simulink model "EPD629_WilliamsJ_AS12"  (R2021b)
settings: Solver=VariableStepAuto  StartTime=0.0  StopTime=45  MaxStep=0.0005  RelTol=1e-3
values from neighbouring files (symbols this model uses):
  AirMassFracO2 = 0.233    [EPD629_HW12_init.m]
  BPVAreaBreakpoints_pct = BPVAreaData_pct    [EPD629_HW12_init.m]
  BPVAreaData_pct = EGRValveAreaData_pct    [EPD629_HW12_init.m]
  BPVPositionBreakpoints_pct = EGRValvePositionBreakpoints_pct    [EPD629_HW12_init.m]
  BPVPositionData_pct = BPVPositionBreakpoints_pct    [EPD629_HW12_init.m]
  BPVWideOpenArea_mm2 = pi * BPVDiameter_mm^2 / 4    (= 7853.98163397)    [EPD629_HW12_init.m]
  CACDischargeCoefficient_frac = 0.7    [EPD629_HW12_init.m]
  CACEffectivenessData_frac = [1 0.95 0.92 0.885 0.87 0.85]    [EPD629_HW12_init.m]
  CACEffectivenessMassFlowBP_gps = [0 50 100 200 300 500]    [EPD629_HW12_init.m]
  CACFlowRestrictionArea_mm2 = 2000    [EPD629_HW12_init.m]
  CACVolume_L = 40    [EPD629_HW12_init.m]
  ClearanceVolumeTotal_L = 8/15    (= 0.533333333333)    [EPD629_HW12_init.m]
  Cp_cmp = 1.004    [EPD629_HW12_init.m]
  Cp_trb = 1.073    [EPD629_HW12_init.m]
  DesiredFuelBreakpoints_mg = 0:20:500    [EPD629_HW12_init.m]
  DischargeCoefficient_frac = 0.7    [EPD629_HW12_init.m]
  EGRCDischargeCoefficient_frac = 0.7    [EPD629_HW12_init.m]
  EGRCEffectivenessData_frac = [1 0.95 0.92 0.885 0.87 0.85]    [EPD629_HW12_init.m]
  EGRCEffectivenessMassFlowBP_gps = [0 50 100 200 300 500]    [EPD629_HW12_init.m]
  EGRCFlowRestrictionArea_mm2 = 500    [EPD629_HW12_init.m]
  EGRCoolerToValveVolume_L = 2    [EPD629_HW12_init.m]
  EGRValveAreaBreakpoints_pct = EGRValveAreaData_pct    [EPD629_HW12_init.m]
  EGRValveAreaData_pct = 100 * EGRValveArea_mm2 / EGRValveWideOpenArea_mm2    [EPD629_HW12_init.m]
  EGRValvePositionBreakpoints_pct = 0:100    [EPD629_HW12_init.m]
  EGRValvePositionData_pct = EGRValvePositionBreakpoints_pct    [EPD629_HW12_init.m]
  EGRValveWideOpenArea_mm2 = pi/4*50^2    (= 1963.49540849)    [EPD629_HW12_init.m]
  EngineDisplacement_L = 8    [EPD629_HW12_init.m]
  EngineSpeedBreakpoints_rpm = 600:200:3000    [EPD629_HW12_init.m]
  ExhaustManifoldGasConstant_kJpkgK = R_trb    (= 0.287)    [EPD629_HW12_init.m]
  ExhaustManifoldVolume_L = 8    [EPD629_HW12_init.m]
  FlowFunctionData_frac = PR.^(1/k_trb) .*      sqrt( 2 * k_trb / (k_trb - 1) .*      (1 - PR.^((k_trb - 1) / k_trb)) )    [EPD629_HW12_init.m]
  IntakeManifoldGasConstant_kJpkgK = Cp_im - Cv_im    (= 0.288)    [EPD629_HW12_init.m]
  IntakeManifoldVolume_L = 8    [EPD629_HW12_init.m]
  k_cmp = Cp_cmp/Cv_cmp    (= 1.40027894003)    [EPD629_HW12_init.m]
  k_trb = Cp_trb/Cv_trb    (= 1.36513994911)    [EPD629_HW12_init.m]
  ManifoldPressureBreakpoints_kPa = 80:20:500    [EPD629_HW12_init.m]
  NumberOfCylinders = 6    [EPD629_HW12_init.m]
  PressureRatioBreakpoints_frac = 0:0.01:1    [EPD629_HW12_init.m]
  R_cmp = Cp_cmp - Cv_cmp    (= 0.287)    [EPD629_HW12_init.m]
  R_trb = Cp_trb - Cv_trb    (= 0.287)    [EPD629_HW12_init.m]
  StoichiometricAFR_frac = 14.7    [EPD629_HW12_init.m]
  TurbineToBPVVolume_L = 10    [EPD629_HW12_init.m]
  TurbochargerInertia_kgm2 = 1e-4    (= 0.0001)    [EPD629_HW12_init.m]
  WastegateAreaData_pct = [0 100]    [EPD629_HW12_init.m]
  WastegateAreaGagePressBreakpoints_kPa = [250 300]    [EPD629_HW12_init.m]
  WastegateWideOpenArea_mm2 = pi/4*20^2    (= 314.159265359)    [EPD629_HW12_init.m]
undefined symbols (not defined in the file or in its folder): APPR_cmp, APPR_trb, ARPM_cmp, ARPM_trb, EFFI_cmp, EFFI_trb, ExhaustTemperatureData_degC, MASS_cmp, MASS_trb, MXRSP_cmp, MXRSP_trb, MXRVOL_cmp, MXRVOL_trb, PMAX_cmp, PMAX_trb, PMIN_cmp, PMIN_trb, ResidualCorrectionFactorData, VolumetricEfficiencyData_frac
libraries: simulink x2
(part 2 of 3)

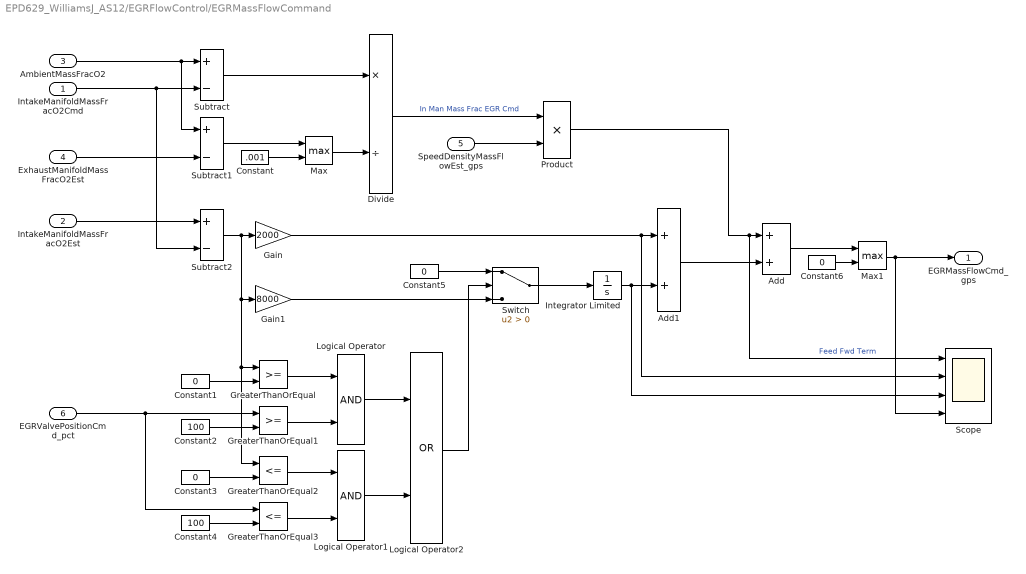
== system EPD629_WilliamsJ_AS12/EGRFlowControl/EGRMassFlowCommand ==
  IntakeManifoldMassFracO2Cmd : Inport
  IntakeManifoldMassFracO2Est : Inport  Port=2
  AmbientMassFracO2 : Inport  Port=3
  ExhaustManifoldMassFracO2Est : Inport  Port=4
  SpeedDensityMassFlowEst_gps : Inport  Port=5
  EGRValvePositionCmd_pct : Inport  Port=6
  Add : Sum
  Add1 : Sum
  Constant : Constant  Value=.001
  Constant{1,3,5..6} (4 alike) : Constant  Value=0
  Constant2 : Constant  Value=100
  Constant4 : Constant  Value=100
  Divide : Product  Inputs=*/
  Gain : Gain  Gain=2000
  Gain1 : Gain  Gain=8000
  GreaterThanOrEqual : RelationalOperator  OutDataTypeStr=boolean  RndMeth=Simplest
  GreaterThanOrEqual1 : RelationalOperator  OutDataTypeStr=boolean  RndMeth=Simplest
  GreaterThanOrEqual2 : RelationalOperator  Operator=<=  OutDataTypeStr=boolean  RndMeth=Simplest
  GreaterThanOrEqual3 : RelationalOperator  Operator=<=  OutDataTypeStr=boolean  RndMeth=Simplest
  Integrator Limited : Integrator  LimitOutput=on  UpperSaturationLimit=20  LowerSaturationLimit=-20
  Logical Operator : Logic  AllPortsSameDT=off  OutDataTypeStr=boolean
  Logical Operator1 : Logic  AllPortsSameDT=off  OutDataTypeStr=boolean
  Logical Operator2 : Logic  Operator=OR  AllPortsSameDT=off  OutDataTypeStr=boolean
  Max : MinMax  Function=max  Inputs=2
  Max1 : MinMax  Function=max  Inputs=2
  Product : Product
  Scope : Scope  NumInputPorts=4
  Subtract : Sum  Inputs=+-
  Subtract1 : Sum  Inputs=+-
  Subtract2 : Sum  Inputs=+-
  Switch : Switch  Criteria=u2 > Threshold
  EGRMassFlowCmd_gps : Outport
  wires:
  AmbientMassFracO2/1 -> Subtract/1, Subtract1/1
  IntakeManifoldMassFracO2Cmd/1 -> Subtract2/2, Subtract/2
  ExhaustManifoldMassFracO2Est/1 -> Subtract1/2
  IntakeManifoldMassFracO2Est/1 -> Subtract2/1
  Constant/1 -> Max/2
  Subtract1/1 -> Max/1
  Subtract/1 -> Divide/1
  Max/1 -> Divide/2
  Divide/1 -> Product/1  "In Man Mass Frac EGR Cmd"
  SpeedDensityMassFlowEst_gps/1 -> Product/2
  Product/1 -> Scope/1, Add/1  "Feed Fwd Term"
  Subtract2/1 -> GreaterThanOrEqual2/1, GreaterThanOrEqual/1, Gain1/1, Gain/1
  Gain/1 -> Scope/2, Add1/1
  Gain1/1 -> Switch/3
  Constant1/1 -> GreaterThanOrEqual/2
  EGRValvePositionCmd_pct/1 -> GreaterThanOrEqual3/1, GreaterThanOrEqual1/1
  Constant2/1 -> GreaterThanOrEqual1/2
  Constant3/1 -> GreaterThanOrEqual2/2
  Constant4/1 -> GreaterThanOrEqual3/2
  GreaterThanOrEqual1/1 -> Logical Operator/2
  GreaterThanOrEqual/1 -> Logical Operator/1
  GreaterThanOrEqual2/1 -> Logical Operator1/1
  GreaterThanOrEqual3/1 -> Logical Operator1/2
  Logical Operator/1 -> Logical Operator2/1
  Logical Operator1/1 -> Logical Operator2/2
  Constant5/1 -> Switch/1
  Logical Operator2/1 -> Switch/2
  Switch/1 -> Integrator Limited/1
  Integrator Limited/1 -> Scope/3, Add1/2
  Add1/1 -> Add/2
  Constant6/1 -> Max1/2
  Add/1 -> Max1/1
  Max1/1 -> Scope/4, EGRMassFlowCmd_gps/1

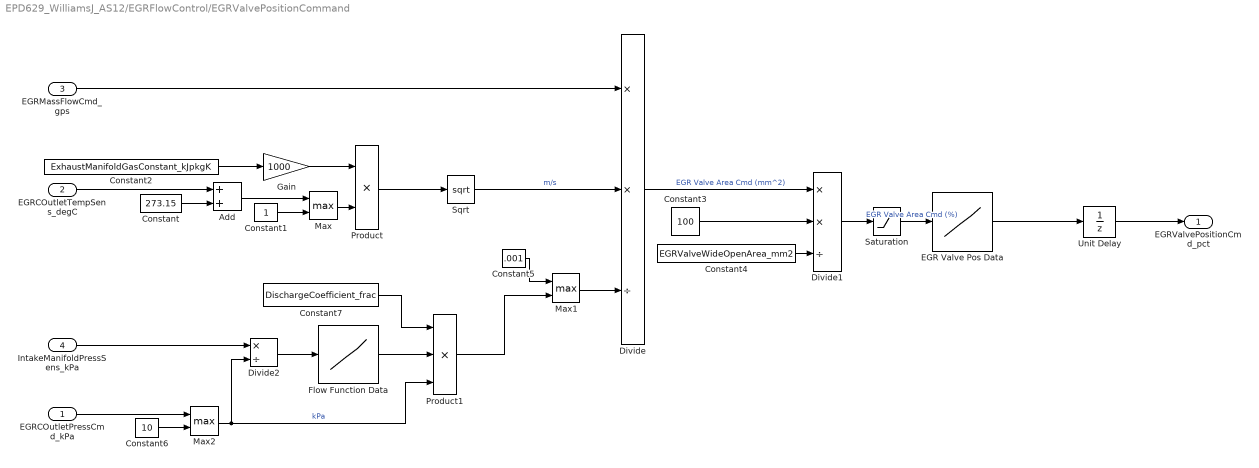
== system EPD629_WilliamsJ_AS12/EGRFlowControl/EGRValvePositionCommand ==
  EGRCOutletPressCmd_kPa : Inport
  EGRCOutletTempSens_degC : Inport  Port=2
  EGRMassFlowCmd_gps : Inport  Port=3
  IntakeManifoldPressSens_kPa : Inport  Port=4
  Add : Sum
  Constant : Constant  Value=273.15
  Constant1 : Constant
  Constant2 : Constant  Value=ExhaustManifoldGasConstant_kJpkgK
  Constant3 : Constant  Value=100
  Constant4 : Constant  Value=EGRValveWideOpenArea_mm2
  Constant5 : Constant  Value=.001
  Constant6 : Constant  Value=10
  Constant7 : Constant  Value=DischargeCoefficient_frac
  Divide : Product  Inputs=**/
  Divide1 : Product  Inputs=**/
  Divide2 : Product  Inputs=*/
  EGR Valve Pos Data : Lookup_n-D  NumberOfTableDimensions=1  BreakpointsForDimension1=EGRValveAreaBreakpoints_pct  Table=EGRValvePositionData_pct  ExtrapMethod=Clip  UseLastTableValue=on  InternalRulePriority=Speed  RndMeth=Simplest  InputSameDT=on
  Flow Function Data : Lookup_n-D  NumberOfTableDimensions=1  BreakpointsForDimension1=PressureRatioBreakpoints_frac  Table=FlowFunctionData_frac  ExtrapMethod=Clip  UseLastTableValue=on  InternalRulePriority=Speed  RndMeth=Simplest  InputSameDT=on
  Gain : Gain  Gain=1000
  Max : MinMax  Function=max  Inputs=2
  Max1 : MinMax  Function=max  Inputs=2
  Max2 : MinMax  Function=max  Inputs=2
  Product : Product
  Product1 : Product  Inputs=3
  Saturation : Saturate  UpperLimit=100  LowerLimit=0
  Sqrt : Sqrt  SaturateOnIntegerOverflow=on
  Unit Delay : UnitDelay  SampleTime=-1  HasFrameUpgradeWarning=on
      settings: AttributesFormatString=IC: %<InitialCondition>
  EGRValvePositionCmd_pct : Outport
  wires:
  Unit Delay/1 -> EGRValvePositionCmd_pct/1
  Constant/1 -> Add/2
  EGRCOutletTempSens_degC/1 -> Add/1
  Add/1 -> Max/1
  Constant1/1 -> Max/2
  Max/1 -> Product/2
  Gain/1 -> Product/1
  Constant2/1 -> Gain/1
  EGRMassFlowCmd_gps/1 -> Divide/1
  Product/1 -> Sqrt/1
  Sqrt/1 -> Divide/2  "m/s"
  Divide/1 -> Divide1/1  "EGR Valve Area Cmd (mm^2)"
  Constant3/1 -> Divide1/2
  Constant4/1 -> Divide1/3
  Divide1/1 -> Saturation/1
  Saturation/1 -> EGR Valve Pos Data/1  "EGR Valve Area Cmd (%)"
  EGR Valve Pos Data/1 -> Unit Delay/1
  Constant5/1 -> Max1/1
  Max1/1 -> Divide/3
  IntakeManifoldPressSens_kPa/1 -> Divide2/1
  Constant6/1 -> Max2/2
  EGRCOutletPressCmd_kPa/1 -> Max2/1
  Max2/1 -> Divide2/2, Product1/3  "kPa"
  Divide2/1 -> Flow Function Data/1
  Flow Function Data/1 -> Product1/2
  Constant7/1 -> Product1/1
  Product1/1 -> Max1/2

== system EPD629_WilliamsJ_AS12/EGRFlowControl/IntakeManifoldMassFractionO2Command ==
  CylinderInMassEst_mg : Inport
  CylinderIVCMassEst_mg : Inport  Port=2
  CylinderIVCMassFracO2Cmd : Inport  Port=3
  CylinderResidualMassO2Est_mg : Inport  Port=4
  Constant : Constant  Value=0
  Constant1 : Constant
  Divide : Product  Inputs=*/
  Max : MinMax  Function=max  Inputs=2
  Max1 : MinMax  Function=max  Inputs=2
  Product : Product
  Subtract : Sum  Inputs=+-
  IntakeManifoldMassFracO2Cmd : Outport
  wires:
  CylinderIVCMassFracO2Cmd/1 -> Product/1
  CylinderIVCMassEst_mg/1 -> Product/2
  Product/1 -> Subtract/1  "Cyl IVC Mass O2 Cmd (mg)"
  CylinderResidualMassO2Est_mg/1 -> Subtract/2
  Subtract/1 -> Max/2
  Constant/1 -> Max/1
  Max/1 -> Divide/1  "Cyl In Mass O2 Cmd (mg)"
  Constant1/1 -> Max1/2
  CylinderInMassEst_mg/1 -> Max1/1
  Max1/1 -> Divide/2
  Divide/1 -> IntakeManifoldMassFracO2Cmd/1

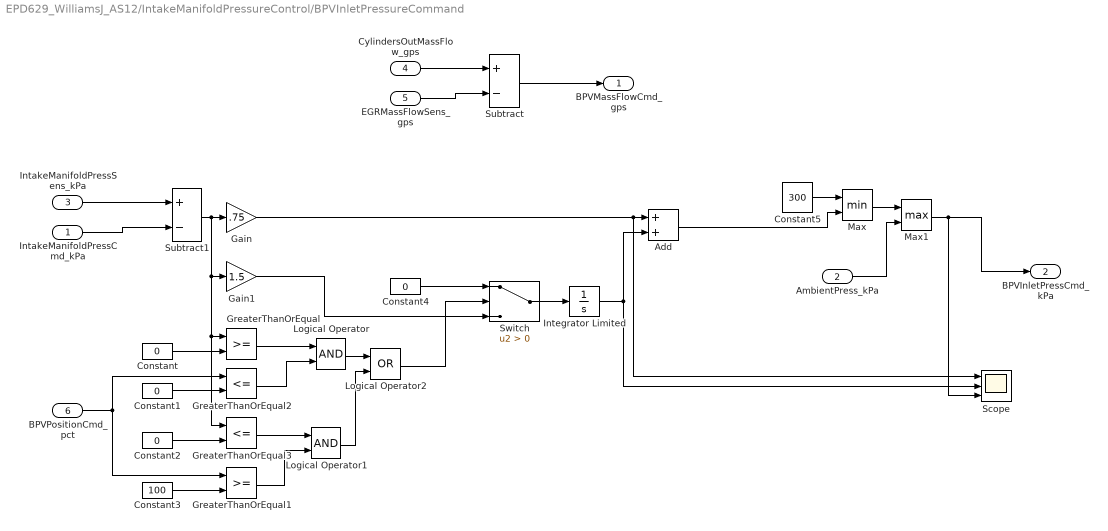
== system EPD629_WilliamsJ_AS12/IntakeManifoldPressureControl/BPVInletPressureCommand ==
  IntakeManifoldPressCmd_kPa : Inport
  AmbientPress_kPa : Inport  Port=2
  IntakeManifoldPressSens_kPa : Inport  Port=3
  CylindersOutMassFlow_gps : Inport  Port=4
  EGRMassFlowSens_gps : Inport  Port=5
  BPVPositionCmd_pct : Inport  Port=6
  Add : Sum
  Constant{,1..2,4} (4 alike) : Constant  Value=0
  Constant3 : Constant  Value=100
  Constant5 : Constant  Value=300
  Gain : Gain  Gain=.75
  Gain1 : Gain  Gain=1.5
  GreaterThanOrEqual : RelationalOperator  OutDataTypeStr=boolean  RndMeth=Simplest
  GreaterThanOrEqual1 : RelationalOperator  OutDataTypeStr=boolean  RndMeth=Simplest
  GreaterThanOrEqual2 : RelationalOperator  Operator=<=  OutDataTypeStr=boolean  RndMeth=Simplest
  GreaterThanOrEqual3 : RelationalOperator  Operator=<=  OutDataTypeStr=boolean  RndMeth=Simplest
  Integrator Limited : Integrator  InitialCondition=100  LimitOutput=on  UpperSaturationLimit=300  LowerSaturationLimit=100
  Logical Operator : Logic  AllPortsSameDT=off  OutDataTypeStr=boolean
  Logical Operator1 : Logic  AllPortsSameDT=off  OutDataTypeStr=boolean
  Logical Operator2 : Logic  Operator=OR  AllPortsSameDT=off  OutDataTypeStr=boolean
  Max : MinMax  Inputs=2
  Max1 : MinMax  Function=max  Inputs=2
  Scope : Scope  NumInputPorts=3
  Subtract : Sum  Inputs=+-
  Subtract1 : Sum  Inputs=+-
  Switch : Switch  Criteria=u2 > Threshold
  BPVMassFlowCmd_gps : Outport
  BPVInletPressCmd_kPa : Outport  Port=2
  wires:
  CylindersOutMassFlow_gps/1 -> Subtract/1
  EGRMassFlowSens_gps/1 -> Subtract/2
  Subtract/1 -> BPVMassFlowCmd_gps/1
  IntakeManifoldPressSens_kPa/1 -> Subtract1/1
  IntakeManifoldPressCmd_kPa/1 -> Subtract1/2
  Subtract1/1 -> GreaterThanOrEqual3/1, GreaterThanOrEqual/1, Gain1/1, Gain/1
  Gain/1 -> Scope/1, Add/1
  Constant/1 -> GreaterThanOrEqual/2
  Constant1/1 -> GreaterThanOrEqual2/2
  BPVPositionCmd_pct/1 -> GreaterThanOrEqual1/1, GreaterThanOrEqual2/1
  Constant2/1 -> GreaterThanOrEqual3/2
  Constant3/1 -> GreaterThanOrEqual1/2
  GreaterThanOrEqual/1 -> Logical Operator/1
  GreaterThanOrEqual2/1 -> Logical Operator/2
  GreaterThanOrEqual3/1 -> Logical Operator1/1
  GreaterThanOrEqual1/1 -> Logical Operator1/2
  Logical Operator/1 -> Logical Operator2/1
  Logical Operator1/1 -> Logical Operator2/2
  Constant4/1 -> Switch/1
  Logical Operator2/1 -> Switch/2
  Gain1/1 -> Switch/3
  Switch/1 -> Integrator Limited/1
  Integrator Limited/1 -> Add/2, Scope/2
  Constant5/1 -> Max/1
  Add/1 -> Max/2
  Max/1 -> Max1/1
  AmbientPress_kPa/1 -> Max1/2
  Max1/1 -> Scope/3, BPVInletPressCmd_kPa/1

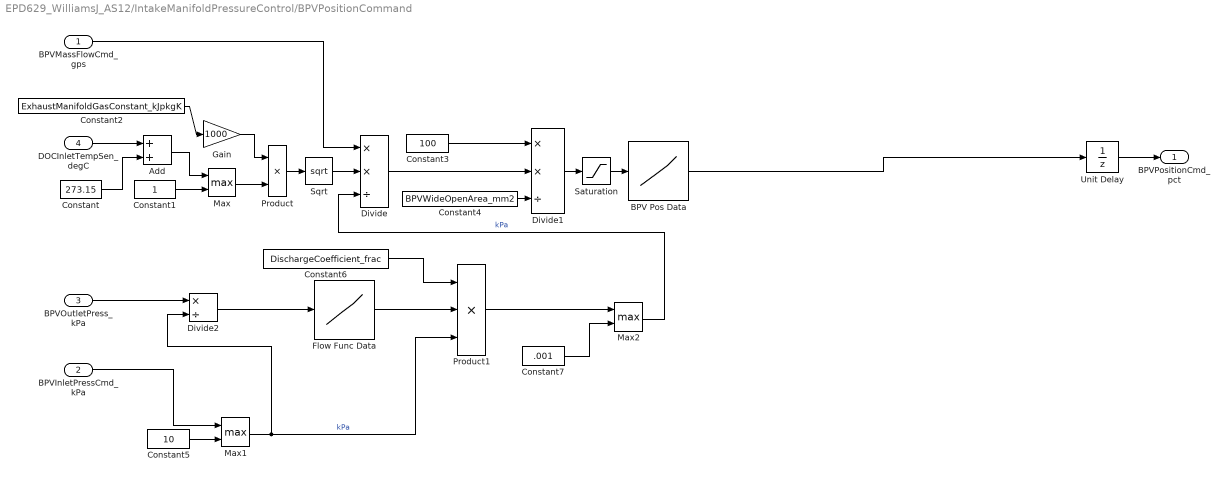
== system EPD629_WilliamsJ_AS12/IntakeManifoldPressureControl/BPVPositionCommand ==
  BPVMassFlowCmd_gps : Inport
  BPVInletPressCmd_kPa : Inport  Port=2
  BPVOutletPress_kPa : Inport  Port=3
  DOCInletTempSen_degC : Inport  Port=4
  Add : Sum
  BPV Pos Data : Lookup_n-D  NumberOfTableDimensions=1  BreakpointsForDimension1=BPVAreaBreakpoints_pct  Table=BPVPositionData_pct  ExtrapMethod=Clip  UseLastTableValue=on  InternalRulePriority=Speed  RndMeth=Simplest  InputSameDT=on
  Constant : Constant  Value=273.15
  Constant1 : Constant
  Constant2 : Constant  Value=ExhaustManifoldGasConstant_kJpkgK
  Constant3 : Constant  Value=100
  Constant4 : Constant  Value=BPVWideOpenArea_mm2
  Constant5 : Constant  Value=10
  Constant6 : Constant  Value=DischargeCoefficient_frac
  Constant7 : Constant  Value=.001
  Divide : Product  Inputs=**/
  Divide1 : Product  Inputs=**/
  Divide2 : Product  Inputs=*/
  Flow Func Data : Lookup_n-D  NumberOfTableDimensions=1  BreakpointsForDimension1=PressureRatioBreakpoints_frac  Table=FlowFunctionData_frac  ExtrapMethod=Clip  UseLastTableValue=on  InternalRulePriority=Speed  RndMeth=Simplest  InputSameDT=on
  Gain : Gain  Gain=1000
  Max : MinMax  Function=max  Inputs=2
  Max1 : MinMax  Function=max  Inputs=2
  Max2 : MinMax  Function=max  Inputs=2
  Product : Product
  Product1 : Product  Inputs=3
  Saturation : Saturate  UpperLimit=100  LowerLimit=0
  Sqrt : Sqrt  SaturateOnIntegerOverflow=on
  Unit Delay : UnitDelay  InitialCondition=100  SampleTime=-1  HasFrameUpgradeWarning=on
      settings: AttributesFormatString=IC: %<InitialCondition>
  BPVPositionCmd_pct : Outport
  wires:
  Unit Delay/1 -> BPVPositionCmd_pct/1
  DOCInletTempSen_degC/1 -> Add/1
  Constant/1 -> Add/2
  Constant1/1 -> Max/2
  Add/1 -> Max/1
  Max/1 -> Product/2
  Gain/1 -> Product/1
  Constant2/1 -> Gain/1
  Product/1 -> Sqrt/1
  Sqrt/1 -> Divide/2
  BPVMassFlowCmd_gps/1 -> Divide/1
  Divide/1 -> Divide1/2
  Constant3/1 -> Divide1/1
  Constant4/1 -> Divide1/3
  Divide1/1 -> Saturation/1
  Saturation/1 -> BPV Pos Data/1
  BPV Pos Data/1 -> Unit Delay/1
  Max1/1 -> Product1/3, Divide2/2  "kPa"
  Constant5/1 -> Max1/2
  BPVInletPressCmd_kPa/1 -> Max1/1
  BPVOutletPress_kPa/1 -> Divide2/1
  Divide2/1 -> Flow Func Data/1
  Flow Func Data/1 -> Product1/2
  Constant6/1 -> Product1/1
  Constant7/1 -> Max2/2
  Product1/1 -> Max2/1
  Max2/1 -> Divide/3  "kPa"

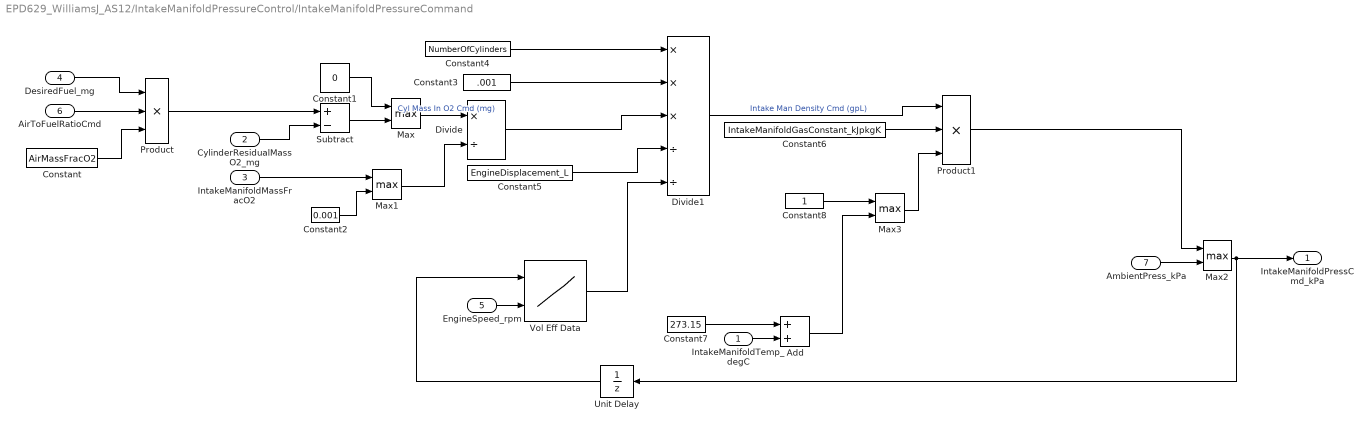
== system EPD629_WilliamsJ_AS12/IntakeManifoldPressureControl/IntakeManifoldPressureCommand ==
  IntakeManifoldTemp_degC : Inport
  CylinderResidualMassO2_mg : Inport  Port=2
  IntakeManifoldMassFracO2 : Inport  Port=3
  DesiredFuel_mg : Inport  Port=4
  EngineSpeed_rpm : Inport  Port=5
  AirToFuelRatioCmd : Inport  Port=6
  AmbientPress_kPa : Inport  Port=7
  Add : Sum
  Constant : Constant  Value=AirMassFracO2
  Constant1 : Constant  Value=0
  Constant2 : Constant  Value=0.001
  Constant3 : Constant  Value=.001
  Constant4 : Constant  Value=NumberOfCylinders
  Constant5 : Constant  Value=EngineDisplacement_L
  Constant6 : Constant  Value=IntakeManifoldGasConstant_kJpkgK
  Constant7 : Constant  Value=273.15
  Constant8 : Constant
  Divide : Product  Inputs=*/
  Divide1 : Product  Inputs=***//
  Max{,1..3} (4 alike) : MinMax  Function=max  Inputs=2
  Product : Product  Inputs=3
  Product1 : Product  Inputs=3
  Subtract : Sum  Inputs=+-
  Unit Delay : UnitDelay  InitialCondition=100  SampleTime=-1  HasFrameUpgradeWarning=on
  Vol Eff Data : Lookup_n-D  BreakpointsForDimension1=ManifoldPressureBreakpoints_kPa  BreakpointsForDimension2=EngineSpeedBreakpoints_rpm  Table=VolumetricEfficiencyData_frac  ExtrapMethod=Clip  UseLastTableValue=on  InternalRulePriority=Speed  RndMeth=Simplest  InputSameDT=on
      settings: InputPortMap=u0,u1
  IntakeManifoldPressCmd_kPa : Outport
  wires:
  DesiredFuel_mg/1 -> Product/1
  AirToFuelRatioCmd/1 -> Product/2
  Constant/1 -> Product/3
  Product/1 -> Subtract/1
  CylinderResidualMassO2_mg/1 -> Subtract/2
  Subtract/1 -> Max/2
  Constant1/1 -> Max/1
  Max/1 -> Divide/1  "Cyl Mass In O2 Cmd (mg)"
  Constant2/1 -> Max1/2
  IntakeManifoldMassFracO2/1 -> Max1/1
  Max1/1 -> Divide/2
  Divide/1 -> Divide1/3
  Constant3/1 -> Divide1/2
  Constant4/1 -> Divide1/1
  Constant5/1 -> Divide1/4
  EngineSpeed_rpm/1 -> Vol Eff Data/2
  Divide1/1 -> Product1/1  "Intake Man Density Cmd (gpL)"
  Constant6/1 -> Product1/2
  Product1/1 -> Max2/1
  AmbientPress_kPa/1 -> Max2/2
  Max2/1 -> Unit Delay/1, IntakeManifoldPressCmd_kPa/1
  Max3/1 -> Product1/3
  IntakeManifoldTemp_degC/1 -> Add/2
  Constant7/1 -> Add/1
  Constant8/1 -> Max3/1
  Add/1 -> Max3/2
  Unit Delay/1 -> Vol Eff Data/1
  Vol Eff Data/1 -> Divide1/5

== system EPD629_WilliamsJ_AS12/VirtualSensor/EngineFlow ==
  ExhaustManifoldPress_kPa : Inport
  DesiredFuel_mg : Inport  Port=2
  EngineSpeed_rpm : Inport  Port=3
  IntakeManifoldPress_kPa : Inport  Port=4
  IntakeManifoldTemp_degC : Inport  Port=5
  IntakeManifoldMassFracO2 : Inport  Port=6
  CylinderEVO : Subsystem
  CylinderIVC : Subsystem
  ExhaustTempAndResidualMass : Subsystem
  SpeedDensityMassFlow : Subsystem
  Unit Delay : UnitDelay  SampleTime=-1  HasFrameUpgradeWarning=on
      settings: AttributesFormatString=IC: %<InitialCondition>
  Unit Delay1 : UnitDelay  SampleTime=-1  HasFrameUpgradeWarning=on
      settings: AttributesFormatString=IC: %<InitialCondition>
  CylindersOutMassFlow_gps : Outport
  CylindersOutMassFracO2 : Outport  Port=2
  CylindersOutTemp_degC : Outport  Port=3
  CylinderInMass_mg : Outport  Port=4
  CylinderIVCMass_mg : Outport  Port=5
  CylinderIVCMassAir_mg : Outport  Port=6
  CylinderIVCMassFracO2 : Outport  Port=7
  CylinderResidualMass_mg : Outport  Port=8
  CylinderResidualMassO2_mg : Outport  Port=9
  SpeedDensityMassFlow_gps : Outport  Port=10
  wires:
  CylinderIVC/2(CylinderIVCMassFracO2) -> CylinderIVCMassFracO2/1
  Unit Delay1/1 -> ExhaustTempAndResidualMass/3(CombustionMassFuel_mg)
  CylinderEVO/3(CombustionMassFuel_mg) -> Unit Delay1/1
  Unit Delay/1 -> CylinderIVC/4(CylindersOutMassFracO2)
  CylinderIVC/4(CylinderIVCMass_mg) -> CylinderIVCMass_mg/1, CylinderEVO/2(CylinderIVCMass_mg)
  CylinderEVO/1(CylindersOutMassFlow_gps) -> CylindersOutMassFlow_gps/1
  CylinderEVO/2(CylindersOutMassFracO2) -> CylindersOutMassFracO2/1, Unit Delay/1
  DesiredFuel_mg/1 -> CylinderEVO/5(DesiredFuel_mg)
  CylinderIVC/3(CylinderIVCMassAir_mg) -> CylinderIVCMassAir_mg/1, CylinderEVO/1(CylinderIVCMassAir_mg)
  IntakeManifoldMassFracO2/1 -> CylinderIVC/2(IntakeManifoldMassFracO2)
  SpeedDensityMassFlow/2(CylinderInMass_mg) -> CylinderInMass_mg/1, CylinderIVC/1(CylinderInMass_mg)
  ExhaustTempAndResidualMass/1(CylinderResidualMass_mg) -> CylinderResidualMass_mg/1, CylinderEVO/4(CylinderResidualMass_mg), CylinderIVC/3(CylinderResidualMass_mg)
  ExhaustTempAndResidualMass/2(CylindersOutTemp_degC) -> CylindersOutTemp_degC/1
  ExhaustManifoldPress_kPa/1 -> ExhaustTempAndResidualMass/2(ExhaustManifoldPress_kPa)
  IntakeManifoldTemp_degC/1 -> SpeedDensityMassFlow/2(IntakeManifoldTemp_degC)
  IntakeManifoldPress_kPa/1 -> SpeedDensityMassFlow/1(IntakeManifoldPress_kPa)
  EngineSpeed_rpm/1 -> SpeedDensityMassFlow/3(EngineSpeed_rpm), ExhaustTempAndResidualMass/1(EngineSpeed_rpm), CylinderEVO/3(EngineSpeed_rpm)
  SpeedDensityMassFlow/1(SpeedDensityMassFlow_gps) -> SpeedDensityMassFlow_gps/1
  CylinderIVC/1(CylinderResidualMassO2_mg) -> CylinderResidualMassO2_mg/1

== system EPD629_WilliamsJ_AS12/VirtualSensor/ExhaustManifoldMassFraction ==
  ExhaustManifoldPressSens_kPa : Inport
  CylindersOutMassFlowEst_gps : Inport  Port=2
  CylindersOutMassFracO2Est : Inport  Port=3
  CylindersOutTempEst_degC : Inport  Port=4
  Add : Sum
  Constant : Constant  Value=0.0005
  Constant1 : Constant  Value=ExhaustManifoldVolume_L
  Constant2 : Constant  Value=ExhaustManifoldGasConstant_kJpkgK
  Constant3 : Constant  Value=273.15
  Divide : Product  Inputs=*/
  Divide1 : Product  Inputs=*/
  Divide2 : Product  Inputs=**/
  Integrator : Integrator  LimitOutput=on  UpperSaturationLimit=1000  LowerSaturationLimit=0
  Product : Product
  Product1 : Product
  Product2 : Product
  Saturation : Saturate  UpperLimit=1000  LowerLimit=0
  Saturation1 : Saturate  UpperLimit=1000  LowerLimit=-100
  Subtract : Sum  Inputs=+-
  Subtract1 : Sum  Inputs=+-
  Subtract2 : Sum  Inputs=+-
  Transfer Fcn : TransferFcn  Denominator=[0.05 1]
  Unit Delay : UnitDelay  SampleTime=-1  HasFrameUpgradeWarning=on
  ExhaustManifoldMassFracO2Est : Outport
  wires:
  CylindersOutMassFlowEst_gps/1 -> Subtract1/1, Product/1
  CylindersOutMassFracO2Est/1 -> Product/2
  Product/1 -> Subtract/1
  Product1/1 -> Subtract/2
  Subtract/1 -> Integrator/1  "dmO2/dt"
  Integrator/1 -> Divide/1  "Exh Man Mass O2 Est (g)"
  Unit Delay/1 -> Subtract2/2
  Subtract1/1 -> Product1/1  "ExhManOutMassFlowEst (gps)"
  Constant/1 -> Divide1/2
  Subtract2/1 -> Divide1/1
  Divide1/1 -> Subtract1/2  "dm/dt"
  ExhaustManifoldPressSens_kPa/1 -> Saturation/1
  Saturation/1 -> Divide2/1
  Constant1/1 -> Divide2/2
  Product2/1 -> Divide2/3
  Constant2/1 -> Product2/1
  CylindersOutTempEst_degC/1 -> Saturation1/1
  Saturation1/1 -> Transfer Fcn/1
  Add/1 -> Product2/2
  Transfer Fcn/1 -> Add/1
  Constant3/1 -> Add/2
  Divide2/1 -> Unit Delay/1, Subtract2/1, Divide/2  "Exhaust Manifold Mass Est (g)"
  Divide/1 -> Product1/2, ExhaustManifoldMassFracO2Est/1

== system EPD629_WilliamsJ_AS12/VirtualSensor/IntakeManifoldMassFraction ==
  IntakeManifoldPressSens_kPa : Inport
  IntakeManifoldTemp_degC : Inport  Port=2
  AmbientMassFracO2 : Inport  Port=3
  EGRMassFlowSens_gps : Inport  Port=4
  ExhaustManifoldMassFracO2Est : Inport  Port=5
  SpeedDensityMassFlowEst_gps : Inport  Port=6
  Add : Sum
  Constant : Constant  Value=0.0005
  Constant1 : Constant  Value=IntakeManifoldVolume_L
  Constant2 : Constant  Value=IntakeManifoldGasConstant_kJpkgK
  Constant3 : Constant  Value=273.15
  Divide : Product  Inputs=*/
  Divide1 : Product  Inputs=*/
  Divide2 : Product  Inputs=**/
  Integrator Limited : Integrator  LimitOutput=on  UpperSaturationLimit=1000  LowerSaturationLimit=0
  Product{,1..3} (4 alike) : Product
  Saturation : Saturate  UpperLimit=1000  LowerLimit=10
  Saturation1 : Saturate  UpperLimit=1000  LowerLimit=-100
  Subtract : Sum  Inputs=+-
  Subtract1 : Sum  Inputs=++-
  Subtract2 : Sum  Inputs=++-
  Unit Delay : UnitDelay  SampleTime=-1  HasFrameUpgradeWarning=on
  IntakeManifoldMassFracO2Est : Outport
  wires:
  Unit Delay/1 -> Subtract/2
  Constant/1 -> Divide/2
  Subtract/1 -> Divide/1
  Divide/1 -> Subtract1/1
  Subtract1/1 -> Product/1
  Product/1 -> Subtract2/1
  AmbientMassFracO2/1 -> Product/2
  EGRMassFlowSens_gps/1 -> Subtract1/3, Product1/1
  ExhaustManifoldMassFracO2Est/1 -> Product1/2
  SpeedDensityMassFlowEst_gps/1 -> Subtract1/2, Product2/1
  Subtract2/1 -> Integrator Limited/1
  Integrator Limited/1 -> Divide1/1  "Intake Manifold Mass O2 Est (g)"
  Product1/1 -> Subtract2/2
  Product2/1 -> Subtract2/3
  Divide1/1 -> Product2/2, IntakeManifoldMassFracO2Est/1
  IntakeManifoldPressSens_kPa/1 -> Saturation/1
  Saturation/1 -> Divide2/1
  Constant1/1 -> Divide2/2
  Constant2/1 -> Product3/1
  IntakeManifoldTemp_degC/1 -> Saturation1/1
  Saturation1/1 -> Add/1
  Add/1 -> Product3/2
  Product3/1 -> Divide2/3
  Constant3/1 -> Add/2
  Divide2/1 -> Unit Delay/1, Subtract/1, Divide1/2

== system EPD629_WilliamsJ_AS12/AirSystemPlantModel/EGRFlow/EGRCooler ==
  ExhaustManifoldPress_kPa : Inport
  ExhaustManifoldTemp_degC : Inport  Port=2
  EGRCOutletPress_kPa : Inport  Port=3
  EGRCOutletTemp_degC : Inport  Port=4
  Add : Sum
  Add1 : Sum
  Constant : Constant  Value=2
  Constant1 : Constant  Value=273.15
  Constant2 : Constant
  Constant3 : Constant  Value=ExhaustManifoldGasConstant_kJpkgK
  Constant4 : Constant  Value=0
  Constant5 : Constant  Value=EGRCDischargeCoefficient_frac
  Constant6 : Constant  Value=EGRCFlowRestrictionArea_mm2
  Constant7 : Constant  Value=.001
  Divide : Product  Inputs=*/
  Gain : Gain  Gain=1000
  Gain1 : Gain  Gain=0.5
  Max : MinMax  Function=max  Inputs=2
  Max1 : MinMax  Function=max  Inputs=2
  Product : Product  Inputs=3
  Product1 : Product
  Product2 : Product  Inputs=4
  Sqrt : Sqrt  SaturateOnIntegerOverflow=on
  Subtract : Sum  Inputs=+-
  EGRCoolerMassFlow_gps : Outport
  wires:
  ExhaustManifoldPress_kPa/1 -> Divide/1, Subtract/1
  EGRCOutletPress_kPa/1 -> Subtract/2
  Subtract/1 -> Gain/1
  Constant/1 -> Product/1
  Gain/1 -> Product/2
  ExhaustManifoldTemp_degC/1 -> Add/1
  EGRCOutletTemp_degC/1 -> Add/2
  Add/1 -> Gain1/1
  Gain1/1 -> Add1/1  "Avg Temp (C)"
  Constant1/1 -> Add1/2
  Add1/1 -> Max/1  "Avg Temp (K)"
  Constant2/1 -> Max/2
  Constant3/1 -> Product1/1
  Max/1 -> Product1/2
  Product1/1 -> Divide/2  "EGR Cooler Density (g/L)"
  Divide/1 -> Product/3
  Max1/1 -> Sqrt/1
  Constant4/1 -> Max1/2
  Product/1 -> Max1/1
  Sqrt/1 -> Product2/4
  Constant5/1 -> Product2/3
  Constant6/1 -> Product2/2
  Constant7/1 -> Product2/1  "g/mg"
  Product2/1 -> EGRCoolerMassFlow_gps/1

== system EPD629_WilliamsJ_AS12/AirSystemPlantModel/EGRFlow/EGRCoolerOutletPressure ==
  EGRCoolerMassFlow_gps : Inport
  EGRValveMassFlow_gps : Inport  Port=2
  EGRCOutletTemp_degC : Inport  Port=3
  Add : Sum
  Constant : Constant  Value=IntakeManifoldGasConstant_kJpkgK
  Constant1 : Constant  Value=273.15
  Constant2 : Constant  Value=EGRCoolerToValveVolume_L
  Divide : Product  Inputs=***/
  Max: 1000 Min: 10 IC: 100 : Integrator  InitialCondition=100  LimitOutput=on  UpperSaturationLimit=1000  LowerSaturationLimit=10
  Saturation : Saturate
  Subtract : Sum  Inputs=+-
  EGRCOutletPress_kPa : Outport
  wires:
  EGRCoolerMassFlow_gps/1 -> Subtract/1
  EGRValveMassFlow_gps/1 -> Subtract/2
  Subtract/1 -> Divide/1
  Constant/1 -> Divide/2
  EGRCOutletTemp_degC/1 -> Saturation/1
  Saturation/1 -> Add/1
  Constant1/1 -> Add/2
  Add/1 -> Divide/3  "EGR Cooler Outlet Temp (K)"
  Constant2/1 -> Divide/4
  Divide/1 -> Max: 1000 Min: 10 IC: 100/1
  Max: 1000 Min: 10 IC: 100/1 -> EGRCOutletPress_kPa/1

== system EPD629_WilliamsJ_AS12/AirSystemPlantModel/EGRFlow/EGRCoolerOutletTemperature ==
  EGRMassFlow_gps : Inport
  ExhaustManifoldTemp_degC : Inport  Port=2
  CoolantTemp_degC : Inport  Port=3
  1-D Lookup Table : Lookup_n-D  NumberOfTableDimensions=1  BreakpointsForDimension1=EGRCEffectivenessMassFlowBP_gps  Table=EGRCEffectivenessData_frac  ExtrapMethod=Clip  UseLastTableValue=on  InternalRulePriority=Speed  RndMeth=Simplest  InputSameDT=on
  Product : Product
  Subtract : Sum  Inputs=+-
  Subtract1 : Sum  Inputs=+-
  EGRCOutletTemp_degC : Outport
  wires:
  EGRMassFlow_gps/1 -> 1-D Lookup Table/1
  Subtract/1 -> Product/1
  ExhaustManifoldTemp_degC/1 -> Subtract/1, Subtract1/1
  1-D Lookup Table/1 -> Product/2
  CoolantTemp_degC/1 -> Subtract/2
  Product/1 -> Subtract1/2
  Subtract1/1 -> EGRCOutletTemp_degC/1

== system EPD629_WilliamsJ_AS12/AirSystemPlantModel/EGRFlow/EGRValve ==
  note: kPa
  note: m/s
  note: N*m/kg
  note: k kg*m/s^2/m^2
  note: m^2/s^2
  note: g*m/s^2/mm^2
  note: K
  IntakeManifoldPress_kPa : Inport
  EGRValvePositionCmd_pct : Inport  Port=2
  EGRCOutletPress_kPa : Inport  Port=3
  EGRCOutletTemp_degC : Inport  Port=4
  Add1 : Sum
  Constant : Constant  Value=273.15
  Constant1 : Constant  Value=DischargeCoefficient_frac
  Constant2 : Constant
  Constant3 : Constant  Value=ExhaustManifoldGasConstant_kJpkgK
  Constant5 : Constant  Value=EGRValveWideOpenArea_mm2
  Constant6 : Constant  Value=100
  EGRValveAreaData_pct Table : Lookup_n-D  NumberOfTableDimensions=1  BreakpointsForDimension1=EGRValvePositionBreakpoints_pct  Table=EGRValveAreaData_pct  ExtrapMethod=Clip  UseLastTableValue=on  InternalRulePriority=Speed  RndMeth=Simplest  InputSameDT=on
  FlowFunctionData_frac Table : Lookup_n-D  NumberOfTableDimensions=1  BreakpointsForDimension1=PressureRatioBreakpoints_frac  Table=FlowFunctionData_frac  ExtrapMethod=Clip  UseLastTableValue=on  InternalRulePriority=Speed  RndMeth=Simplest  InputSameDT=on
  Math Function : Math  Operator=sqrt  SignedPower=on  SaturateOnIntegerOverflow=on
  Max2 : MinMax  Function=max  Inputs=2
  Product : Product  Inputs=**/
  Product1 : Product  Inputs=****/  SaturateOnIntegerOverflow=on  OutDataTypeStr=Inherit: Same as first input
  Product2 : Product  Inputs=*/  SaturateOnIntegerOverflow=on  OutDataTypeStr=Inherit: Same as first input
  Product3 : Product  SaturateOnIntegerOverflow=on  OutDataTypeStr=Inherit: Same as first input
  Transfer Fcn : TransferFcn  Denominator=[0.05 1]
  kJ/(kg*K) to J/(kg*K) : Gain  Gain=1000
  EGRValveMassFlow_gps : Outport
  wires:
  Constant5/1 -> Product/2
  Add1/1 -> Max2/1
  Constant1/1 -> Product1/2
  EGRValveAreaData_pct Table/1 -> Product/1  "EGRValveArea_pct"
  Product/1 -> Product1/1  "ThrottleArea_mm2"
  Constant3/1 -> kJ/(kg*K) to J/(kg*K)/1
  EGRCOutletPress_kPa/1 -> Product1/4, Product2/2
  Product3/1 -> Math Function/1
  EGRValvePositionCmd_pct/1 -> Transfer Fcn/1
  FlowFunctionData_frac Table/1 -> Product1/3
  kJ/(kg*K) to J/(kg*K)/1 -> Product3/1
  Math Function/1 -> Product1/5
  Product2/1 -> FlowFunctionData_frac Table/1  "EGRValvePressRatio_frac"
  Max2/1 -> Product3/2
  Constant2/1 -> Max2/2
  IntakeManifoldPress_kPa/1 -> Product2/1
  Constant6/1 -> Product/3
  EGRCOutletTemp_degC/1 -> Add1/1
  Constant/1 -> Add1/2
  Product1/1 -> EGRValveMassFlow_gps/1
  Transfer Fcn/1 -> EGRValveAreaData_pct Table/1

== system EPD629_WilliamsJ_AS12/AirSystemPlantModel/EngineFlow/CylinderEVO ==
  CylinderIVCMassAir_mg : Inport
  CylinderIVCMass_mg : Inport  Port=2
  EngineSpeed_rpm : Inport  Port=3
  CylinderResidualMass_mg : Inport  Port=4
  DesiredFuel_mg : Inport  Port=5
  Add : Sum
  Constant : Constant  Value=StoichiometricAFR_frac
  Constant1 : Constant  Value=AirMassFracO2
  Constant2 : Constant
  Constant3 : Constant  Value=NumberOfCylinders
  Constant4 : Constant  Value=120000
  Divide : Product  Inputs=*/
  Divide1 : Product  Inputs=*/
  Divide2 : Product  Inputs=***/
  Max : MinMax  Function=max  Inputs=2
  Min : MinMax  Inputs=2
  Product : Product
  Product1 : Product
  Subtract : Sum  Inputs=+-
  Subtract1 : Sum  Inputs=+-
  CylindersOutMassFlow_gps : Outport
  CylindersOutMassFracO2 : Outport  Port=2
  CombustionMassFuel_mg : Outport  Port=3
  wires:
  Constant/1 -> Product/2, Divide/2
  CylinderIVCMass_mg/1 -> Add/2
  DesiredFuel_mg/1 -> Min/1, Add/1
  CylinderIVCMassAir_mg/1 -> Divide/1, Subtract/1
  Divide/1 -> Min/2
  Min/1 -> Product/1, CombustionMassFuel_mg/1
  Add/1 -> Max/2, Subtract1/1
  Product/1 -> Subtract/2
  Constant1/1 -> Product1/2
  Subtract/1 -> Product1/1
  Product1/1 -> Divide1/1
  Max/1 -> Divide1/2
  Constant2/1 -> Max/1
  CylinderResidualMass_mg/1 -> Subtract1/2
  Subtract1/1 -> Divide2/1
  EngineSpeed_rpm/1 -> Divide2/2
  Constant3/1 -> Divide2/3
  Constant4/1 -> Divide2/4
  Divide2/1 -> CylindersOutMassFlow_gps/1
  Divide1/1 -> CylindersOutMassFracO2/1

== system EPD629_WilliamsJ_AS12/AirSystemPlantModel/EngineFlow/CylinderIVC ==
  CylinderInMass_mg : Inport
  IntakeManifoldMassFracO2 : Inport  Port=2
  CylinderResidualMass_mg : Inport  Port=3
  CylindersOutMassFracO2 : Inport  Port=4
  Add : Sum
  Add1 : Sum
  Constant : Constant  Value=AirMassFracO2
  Constant1 : Constant
  Divide : Product  Inputs=*/
  Divide1 : Product  Inputs=*/
  Max : MinMax  Function=max  Inputs=2
  Product : Product
  Product1 : Product
  CylinderResidualMassO2_mg : Outport
  CylinderIVCMassFracO2 : Outport  Port=2
  CylinderIVCMassAir_mg : Outport  Port=3
  CylinderIVCMass_mg : Outport  Port=4
  wires:
  CylinderResidualMass_mg/1 -> Add1/2, Product/1
  CylindersOutMassFracO2/1 -> Product/2
  Product/1 -> Add/1  "Cyl Residual Mass O2_mg"
  CylinderInMass_mg/1 -> Add1/1, Product1/1
  IntakeManifoldMassFracO2/1 -> Product1/2
  Product1/1 -> Add/2  "Cyl In Mass O2_mg"
  Add1/1 -> Max/2, CylinderIVCMass_mg/1
  Add/1 -> Divide1/1, Divide/1
  Constant/1 -> Divide/2
  Constant1/1 -> Max/1
  Max/1 -> Divide1/2
  Divide1/1 -> CylinderIVCMassFracO2/1
  Divide/1 -> CylinderIVCMassAir_mg/1

== system EPD629_WilliamsJ_AS12/AirSystemPlantModel/EngineFlow/ExhaustTempAndResidualMass ==
  EngineSpeed_rpm : Inport
  ExhaustManifoldPress_kPa : Inport  Port=2
  CombustionMassFuel_mg : Inport  Port=3
  Add : Sum
  Constant : Constant  Value=ExhaustManifoldGasConstant_kJpkgK
  Constant1 : Constant  Value=273.15
  Constant2 : Constant
  Constant3 : Constant  Value=1000
  Constant4 : Constant  Value=ClearanceVolumeTotal_L
  Constant5 : Constant  Value=NumberOfCylinders
  Divide : Product  Inputs=*//
  Divide1 : Product  Inputs=****/
  Exhaust TEmp Data Table : Lookup_n-D  BreakpointsForDimension1=DesiredFuelBreakpoints_mg  BreakpointsForDimension2=EngineSpeedBreakpoints_rpm  Table=ExhaustTemperatureData_degC  ExtrapMethod=Clip  UseLastTableValue=on  InternalRulePriority=Speed  RndMeth=Simplest  InputSameDT=on
      settings: InputPortMap=u0,u1
  Max : MinMax  Function=max  Inputs=2
  Residual Correction Factor : Lookup_n-D  BreakpointsForDimension1=DesiredFuelBreakpoints_mg  BreakpointsForDimension2=EngineSpeedBreakpoints_rpm  Table=ResidualCorrectionFactorData  ExtrapMethod=Clip  UseLastTableValue=on  InternalRulePriority=Speed  RndMeth=Simplest  InputSameDT=on
      settings: InputPortMap=u0,u1
  CylinderResidualMass_mg : Outport
  CylindersOutTemp_degC : Outport  Port=2
  wires:
  ExhaustManifoldPress_kPa/1 -> Divide/1
  Constant/1 -> Divide/2
  Constant1/1 -> Add/1
  EngineSpeed_rpm/1 -> Residual Correction Factor/2, Exhaust TEmp Data Table/2
  CombustionMassFuel_mg/1 -> Residual Correction Factor/1, Exhaust TEmp Data Table/1
  Exhaust TEmp Data Table/1 -> CylindersOutTemp_degC/1, Add/2
  Add/1 -> Max/1
  Constant2/1 -> Max/2
  Max/1 -> Divide/3
  Divide/1 -> Divide1/2
  Constant3/1 -> Divide1/1
  Constant4/1 -> Divide1/3
  Constant5/1 -> Divide1/5
  Residual Correction Factor/1 -> Divide1/4
  Divide1/1 -> CylinderResidualMass_mg/1

== system EPD629_WilliamsJ_AS12/AirSystemPlantModel/EngineFlow/SpeedDensityMassFlow ==
  note: g
  note: mg/g
  note: K
  note: kg/m^3
      | g/L
  note: kJ/(kg*K)
  note: L
  note: kPa
  IntakeManifoldPress_kPa : Inport
  IntakeManifoldTemp_degC : Inport  Port=2
  EngineSpeed_rpm : Inport  Port=3
  Add1 : Sum
  Constant : Constant  Value=273.15
  Constant2 : Constant  Value=IntakeManifoldGasConstant_kJpkgK
  Constant3 : Constant  Value=EngineDisplacement_L
  Constant4 : Constant
  Constant7 : Constant  Value=NumberOfCylinders
  Max2 : MinMax  Function=max  Inputs=2
  P_a3 : Constant  Value=1000
  Product1 : Product  Inputs=*//  RndMeth=Zero
  Product2 : Product  Inputs=3  RndMeth=Zero
  Product3 : Product
  Product4 : Product  Inputs=**/
  VolumetricEfficiencyData_frac : Lookup_n-D  BreakpointsForDimension1=ManifoldPressureBreakpoints_kPa  BreakpointsForDimension2=EngineSpeedBreakpoints_rpm  Table=VolumetricEfficiencyData_frac  ExtrapMethod=Clip  UseLastTableValue=on  InternalRulePriority=Speed  RndMeth=Simplest  InputSameDT=on
      settings: InputPortMap=u0,u1
  rpm to cycles/sec : Gain  Gain=1/120
  SpeedDensityMassFlow_gps : Outport
  CylinderInMass_mg : Outport  Port=2
  wires:
  Product3/1 -> SpeedDensityMassFlow_gps/1
  Product2/1 -> Product4/2, Product3/2
  Constant7/1 -> Product4/3
  Product4/1 -> CylinderInMass_mg/1
  P_a3/1 -> Product4/1
  Constant2/1 -> Product1/2
  VolumetricEfficiencyData_frac/1 -> Product2/3  "VolumetricEfficiency_frac"
  Constant4/1 -> Max2/2
  Add1/1 -> Max2/1
  IntakeManifoldTemp_degC/1 -> Add1/1
  IntakeManifoldPress_kPa/1 -> VolumetricEfficiencyData_frac/1, Product1/1
  Constant3/1 -> Product2/2
  rpm to cycles/sec/1 -> Product3/1
  Max2/1 -> Product1/3
  Product1/1 -> Product2/1  "IntakeManifoldDensity_gpL"
  Constant/1 -> Add1/2
  EngineSpeed_rpm/1 -> VolumetricEfficiencyData_frac/2, rpm to cycles/sec/1

== system EPD629_WilliamsJ_AS12/AirSystemPlantModel/TurbochargerFlow/CompressorPower ==
  CompressorInletTemp_degC : Inport
  PressureRatio : Inport  Port=2
  Efficiency_frac : Inport  Port=3
  MassFlow_gps : Inport  Port=4
  Add : Sum
  Add1 : Sum
  Add2 : Sum  Inputs=+-
  C to K Constant : Constant  Value=273.15
  C to K Constant1 : Constant
  Constant : Constant  Value=0
  Constant1 : Constant  Value=.001
  Constant2 : Constant  Value=k_cmp
  Constant3 : Constant  Value=.001
  Constant4 : Constant
  Constant5 : Constant  Value=Cp_cmp
  Constant6 : Constant  Value=.001
  Divide : Product  Inputs=**/
  Divide by Zero Protection : MinMax  Function=max  Inputs=2
  Divide1 : Product  Inputs=*/
  Max : MinMax  Function=max  Inputs=2
  Max1 : MinMax  Function=max  Inputs=2
  Max: 2000 Min: -100 : Saturate  UpperLimit=2000  LowerLimit=-100
  Power : Math  Operator=pow  SaturateOnIntegerOverflow=on
  Product : Product  Inputs=4
  Subtract : Sum  Inputs=+-
  CompressorOutletTemp_degC : Outport
  CompressorPower_kW : Outport  Port=2
  wires:
  CompressorInletTemp_degC/1 -> Add1/1, Add/1
  C to K Constant/1 -> Add/2
  Add/1 -> Max/1  "Temp (K)"
  Constant/1 -> Max/2
  Max/1 -> Divide/1
  Constant1/1 -> Max1/2
  PressureRatio/1 -> Max1/1
  Max1/1 -> Power/1
  C to K Constant1/1 -> Add2/2
  Constant2/1 -> Add2/1, Divide1/2
  Add2/1 -> Divide1/1  "Temp (K)"
  Divide1/1 -> Power/2
  Efficiency_frac/1 -> Divide by Zero Protection/1
  Constant3/1 -> Divide by Zero Protection/2
  Power/1 -> Subtract/1
  Constant4/1 -> Subtract/2
  Subtract/1 -> Divide/2
  Divide by Zero Protection/1 -> Divide/3
  Divide/1 -> Product/4, Add1/2
  MassFlow_gps/1 -> Product/2  "g/s"
  Constant5/1 -> Product/3
  Constant6/1 -> Product/1  "kW/W"
  Product/1 -> CompressorPower_kW/1
  Max: 2000 Min: -100/1 -> CompressorOutletTemp_degC/1
  Add1/1 -> Max: 2000 Min: -100/1

== system EPD629_WilliamsJ_AS12/AirSystemPlantModel/TurbochargerFlow/CompressorPressureRatio ==
  note: divide by zero
      | protection
  CompressorOutletPress_kPa : Inport
  CompressorInletPress_kPa : Inport  Port=2
  Constant4 : Constant
  Max : MinMax  Function=max  Inputs=2
  Product3 : Product  Inputs=*/
  CompressorPressureRatio : Outport
  wires:
  Constant4/1 -> Max/2
  Max/1 -> Product3/2
  CompressorInletPress_kPa/1 -> Max/1
  CompressorOutletPress_kPa/1 -> Product3/1
  Product3/1 -> CompressorPressureRatio/1

== system EPD629_WilliamsJ_AS12/AirSystemPlantModel/TurbochargerFlow/TurbinePower ==
  TurbineInletTemp_degC : Inport
  PressureRatio : Inport  Port=2
  Efficiency_frac : Inport  Port=3
  MassFlow_gps : Inport  Port=4
  Add : Sum
  Add1 : Sum  Inputs=+-
  Add2 : Sum  Inputs=+-
  C to K Constant : Constant  Value=273.15
  C to K Constant1 : Constant
  Constant : Constant  Value=0
  Constant1 : Constant  Value=.001
  Constant2 : Constant  Value=k_trb
  Constant4 : Constant
  Constant5 : Constant  Value=Cp_trb
  Constant6 : Constant  Value=.001
  Divide : Product  Inputs=***
  Divide1 : Product  Inputs=*/
  Max : MinMax  Function=max  Inputs=2
  Max1 : MinMax  Function=max  Inputs=2
  Max: 2000 Min: -100 : Saturate  UpperLimit=2000  LowerLimit=-100
  Power : Math  Operator=pow  SaturateOnIntegerOverflow=on
  Product : Product  Inputs=4
  Subtract : Sum  Inputs=+-
  TurbinePower_kW : Outport
  TurbineOutletTemp_degC : Outport  Port=2
  wires:
  Efficiency_frac/1 -> Divide/3
  Product/1 -> TurbinePower_kW/1
  Subtract/1 -> Divide/2
  Add1/1 -> Max: 2000 Min: -100/1
  Power/1 -> Subtract/2
  Constant5/1 -> Product/3
  Divide1/1 -> Power/2
  PressureRatio/1 -> Max1/1
  Constant/1 -> Max/2
  C to K Constant/1 -> Add/2
  Add/1 -> Max/1  "Temp (K)"
  Constant6/1 -> Product/1  "kW/W"
  MassFlow_gps/1 -> Product/2  "g/s"
  Add2/1 -> Divide1/1  "Temp (K)"
  TurbineInletTemp_degC/1 -> Add/1, Add1/1
  Divide/1 -> Add1/2, Product/4
  Constant1/1 -> Max1/2
  C to K Constant1/1 -> Add2/1
  Max1/1 -> Power/1
  Max/1 -> Divide/1
  Constant4/1 -> Subtract/1
  Constant2/1 -> Add2/2, Divide1/2
  Max: 2000 Min: -100/1 -> TurbineOutletTemp_degC/1

== system EPD629_WilliamsJ_AS12/AirSystemPlantModel/TurbochargerFlow/TurbinePressureRatio ==
  note: divide by zero
      | protection
  TurbineOutletPress_kPa : Inport
  TurbineInletPress_kPa : Inport  Port=2
  Constant4 : Constant
  Max : MinMax  Function=max  Inputs=2
  Product3 : Product  Inputs=*/
  TurbinePressureRatio : Outport
  wires:
  Product3/1 -> TurbinePressureRatio/1
  TurbineInletPress_kPa/1 -> Product3/1
  TurbineOutletPress_kPa/1 -> Max/1
  Max/1 -> Product3/2
  Constant4/1 -> Max/2

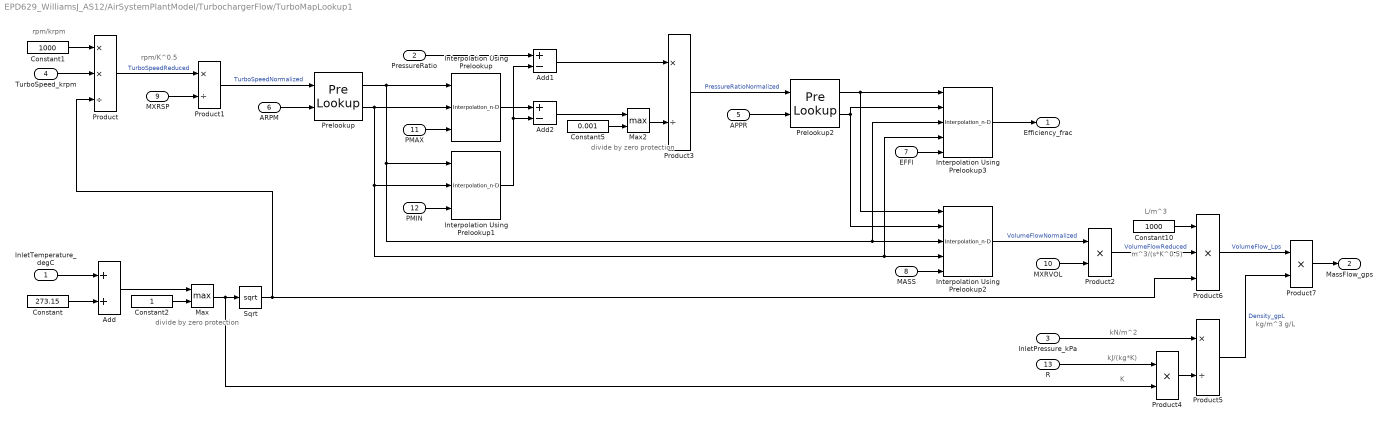
== system EPD629_WilliamsJ_AS12/AirSystemPlantModel/TurbochargerFlow/TurboMapLookup1 ==
  note: rpm/krpm
  note: kg/m^3
      | g/L
  note: L/m^3
  note: m^3/(s*K^0.5)
  note: kN/m^2
  note: kJ/(kg*K)
  note: K
  note: rpm/K^0.5
  note: divide by zero
      | protection
  note: divide by zero
      | protection
  InletTemperature_degC : Inport
  PressureRatio : Inport  Port=2
  InletPressure_kPa : Inport  Port=3
  TurboSpeed_krpm : Inport  Port=4
  APPR : Inport  Port=5
  ARPM : Inport  Port=6
  EFFI : Inport  Port=7
  MASS : Inport  Port=8
  MXRSP : Inport  Port=9
  MXRVOL : Inport  Port=10
  PMAX : Inport  Port=11
  PMIN : Inport  Port=12
  R : Inport  Port=13
  Add : Sum
  Add1 : Sum  Inputs=+-
  Add2 : Sum  Inputs=+-
  Constant : Constant  Value=273.15
  Constant1 : Constant  Value=1000
  Constant10 : Constant  Value=1000
  Constant2 : Constant
  Constant5 : Constant  Value=0.001
  Interpolation Using Prelookup : Interpolation_n-D  NumberOfTableDimensions=1  TableSource=Input port  ExtrapMethod=Clip  ValidIndexMayReachLast=on  InternalRulePriority=Speed
      settings: InputPortMap=u0,u1,p2
  Interpolation Using Prelookup1 : Interpolation_n-D  NumberOfTableDimensions=1  TableSource=Input port  ExtrapMethod=Clip  ValidIndexMayReachLast=on  InternalRulePriority=Speed
      settings: InputPortMap=u0,u1,p2
  Interpolation Using Prelookup2 : Interpolation_n-D  TableSource=Input port  ExtrapMethod=Clip  ValidIndexMayReachLast=on  InternalRulePriority=Speed
      settings: InputPortMap=u0,u1,u2,u3,p2
  Interpolation Using Prelookup3 : Interpolation_n-D  TableSource=Input port  ExtrapMethod=Clip  ValidIndexMayReachLast=on  InternalRulePriority=Speed
      settings: InputPortMap=u0,u1,u2,u3,p2
  Max : MinMax  Function=max  Inputs=2
  Max2 : MinMax  Function=max  Inputs=2
  Prelookup : PreLookup  BreakpointsDataSource=Input port  BreakpointsData=[10:10:110]  UseLastBreakpoint=on
      settings: InputPortMap=u0,p1
  Prelookup2 : PreLookup  BreakpointsDataSource=Input port  BreakpointsData=[10:10:110]  UseLastBreakpoint=on
      settings: InputPortMap=u0,p1
  Product : Product  Inputs=**/
  Product1 : Product  Inputs=*/
  Product2 : Product
  Product3 : Product  Inputs=*/
  Product4 : Product
  Product5 : Product  Inputs=*/
  Product6 : Product  Inputs=3
  Product7 : Product
  Sqrt : Sqrt  SaturateOnIntegerOverflow=on
  Efficiency_frac : Outport
  MassFlow_gps : Outport  Port=2
  wires:
  Constant/1 -> Add/2
  InletTemperature_degC/1 -> Add/1
  Product/1 -> Product1/1  "TurboSpeedReduced"
  Constant2/1 -> Max/2
  Add/1 -> Max/1
  Sqrt/1 -> Product6/3, Product/3
  Product1/1 -> Prelookup/1  "TurboSpeedNormalized"
  Max2/1 -> Product3/2
  Constant5/1 -> Max2/2
  Add2/1 -> Max2/1
  Add1/1 -> Product3/1
  Interpolation Using Prelookup1/1 -> Add1/2, Add2/2
  Interpolation Using Prelookup/1 -> Add2/1
  Product3/1 -> Prelookup2/1  "PressureRatioNormalized"
  Interpolation Using Prelookup2/1 -> Product2/1  "VolumeFlowNormalized"
  MXRVOL/1 -> Product2/2
  InletPressure_kPa/1 -> Product5/1
  R/1 -> Product4/1
  PressureRatio/1 -> Add1/1
  Product2/1 -> Product6/2  "VolumeFlowReduced"
  Constant10/1 -> Product6/1
  Product6/1 -> Product7/1  "VolumeFlow_Lps"
  Max/1 -> Product4/2, Sqrt/1
  Product4/1 -> Product5/2
  Product5/1 -> Product7/2  "Density_gpL"
  Product7/1 -> MassFlow_gps/1
  Constant1/1 -> Product/1
  TurboSpeed_krpm/1 -> Product/2
  PMAX/1 -> Interpolation Using Prelookup/3
  PMIN/1 -> Interpolation Using Prelookup1/3
  Prelookup/2 -> Interpolation Using Prelookup3/4, Interpolation Using Prelookup2/4, Interpolation Using Prelookup1/2, Interpolation Using Prelookup/2
  Prelookup/1 -> Interpolation Using Prelookup3/3, Interpolation Using Prelookup2/3, Interpolation Using Prelookup1/1, Interpolation Using Prelookup/1
  MXRSP/1 -> Product1/2
  ARPM/1 -> Prelookup/2
  MASS/1 -> Interpolation Using Prelookup2/5
  Prelookup2/2 -> Interpolation Using Prelookup3/2, Interpolation Using Prelookup2/2
  Prelookup2/1 -> Interpolation Using Prelookup2/1, Interpolation Using Prelookup3/1
  EFFI/1 -> Interpolation Using Prelookup3/5
  Interpolation Using Prelookup3/1 -> Efficiency_frac/1
  APPR/1 -> Prelookup2/2

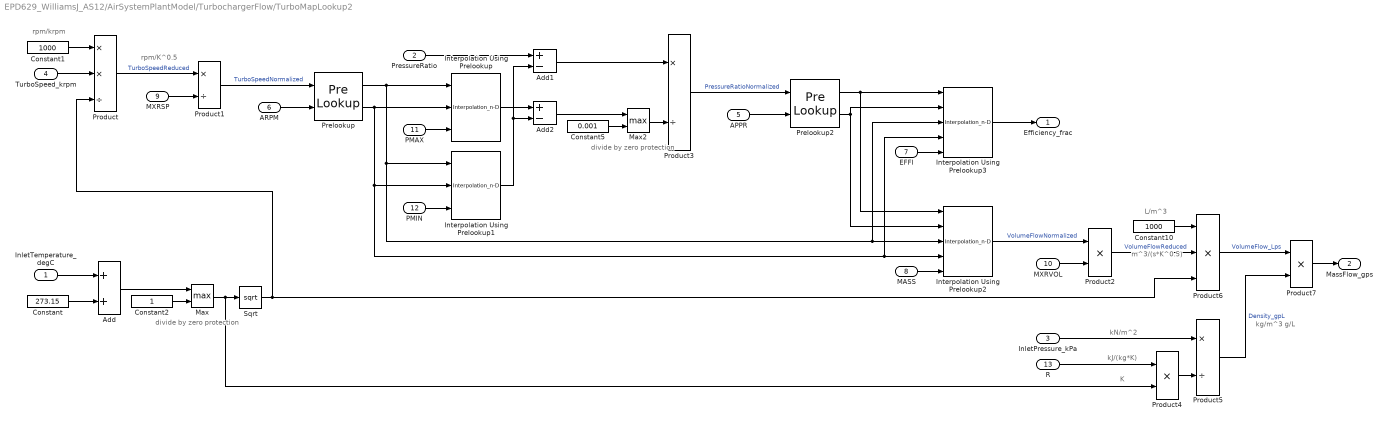
== system EPD629_WilliamsJ_AS12/AirSystemPlantModel/TurbochargerFlow/TurboMapLookup2 ==
  note: divide by zero
      | protection
  note: divide by zero
      | protection
  note: rpm/K^0.5
  note: K
  note: kJ/(kg*K)
  note: kN/m^2
  note: m^3/(s*K^0.5)
  note: L/m^3
  note: kg/m^3
      | g/L
  note: rpm/krpm
  InletTemperature_degC : Inport
  PressureRatio : Inport  Port=2
  InletPressure_kPa : Inport  Port=3
  TurboSpeed_krpm : Inport  Port=4
  APPR : Inport  Port=5
  ARPM : Inport  Port=6
  EFFI : Inport  Port=7
  MASS : Inport  Port=8
  MXRSP : Inport  Port=9
  MXRVOL : Inport  Port=10
  PMAX : Inport  Port=11
  PMIN : Inport  Port=12
  R : Inport  Port=13
  Add : Sum
  Add1 : Sum  Inputs=+-
  Add2 : Sum  Inputs=+-
  Constant : Constant  Value=273.15
  Constant1 : Constant  Value=1000
  Constant10 : Constant  Value=1000
  Constant2 : Constant
  Constant5 : Constant  Value=0.001
  Interpolation Using Prelookup : Interpolation_n-D  NumberOfTableDimensions=1  TableSource=Input port  ExtrapMethod=Clip  ValidIndexMayReachLast=on  InternalRulePriority=Speed
      settings: InputPortMap=u0,u1,p2
  Interpolation Using Prelookup1 : Interpolation_n-D  NumberOfTableDimensions=1  TableSource=Input port  ExtrapMethod=Clip  ValidIndexMayReachLast=on  InternalRulePriority=Speed
      settings: InputPortMap=u0,u1,p2
  Interpolation Using Prelookup2 : Interpolation_n-D  TableSource=Input port  ExtrapMethod=Clip  ValidIndexMayReachLast=on  InternalRulePriority=Speed
      settings: InputPortMap=u0,u1,u2,u3,p2
  Interpolation Using Prelookup3 : Interpolation_n-D  TableSource=Input port  ExtrapMethod=Clip  ValidIndexMayReachLast=on  InternalRulePriority=Speed
      settings: InputPortMap=u0,u1,u2,u3,p2
  Max : MinMax  Function=max  Inputs=2
  Max2 : MinMax  Function=max  Inputs=2
  Prelookup : PreLookup  BreakpointsDataSource=Input port  BreakpointsData=[10:10:110]  UseLastBreakpoint=on
      settings: InputPortMap=u0,p1
  Prelookup2 : PreLookup  BreakpointsDataSource=Input port  BreakpointsData=[10:10:110]  UseLastBreakpoint=on
      settings: InputPortMap=u0,p1
  Product : Product  Inputs=**/
  Product1 : Product  Inputs=*/
  Product2 : Product
  Product3 : Product  Inputs=*/
  Product4 : Product
  Product5 : Product  Inputs=*/
  Product6 : Product  Inputs=3
  Product7 : Product
  Sqrt : Sqrt  SaturateOnIntegerOverflow=on
  Efficiency_frac : Outport
  MassFlow_gps : Outport  Port=2
  wires:
  APPR/1 -> Prelookup2/2
  Interpolation Using Prelookup3/1 -> Efficiency_frac/1
  EFFI/1 -> Interpolation Using Prelookup3/5
  Prelookup2/1 -> Interpolation Using Prelookup3/1, Interpolation Using Prelookup2/1
  Prelookup2/2 -> Interpolation Using Prelookup2/2, Interpolation Using Prelookup3/2
  MASS/1 -> Interpolation Using Prelookup2/5
  ARPM/1 -> Prelookup/2
  MXRSP/1 -> Product1/2
  Prelookup/1 -> Interpolation Using Prelookup/1, Interpolation Using Prelookup1/1, Interpolation Using Prelookup2/3, Interpolation Using Prelookup3/3
  Prelookup/2 -> Interpolation Using Prelookup/2, Interpolation Using Prelookup1/2, Interpolation Using Prelookup2/4, Interpolation Using Prelookup3/4
  PMIN/1 -> Interpolation Using Prelookup1/3
  PMAX/1 -> Interpolation Using Prelookup/3
  TurboSpeed_krpm/1 -> Product/2
  Constant1/1 -> Product/1
  Product7/1 -> MassFlow_gps/1
  Product5/1 -> Product7/2  "Density_gpL"
  Product4/1 -> Product5/2
  Max/1 -> Sqrt/1, Product4/2
  Product6/1 -> Product7/1  "VolumeFlow_Lps"
  Constant10/1 -> Product6/1
  Product2/1 -> Product6/2  "VolumeFlowReduced"
  PressureRatio/1 -> Add1/1
  R/1 -> Product4/1
  InletPressure_kPa/1 -> Product5/1
  MXRVOL/1 -> Product2/2
  Interpolation Using Prelookup2/1 -> Product2/1  "VolumeFlowNormalized"
  Product3/1 -> Prelookup2/1  "PressureRatioNormalized"
  Interpolation Using Prelookup/1 -> Add2/1
  Interpolation Using Prelookup1/1 -> Add2/2, Add1/2
  Add1/1 -> Product3/1
  Add2/1 -> Max2/1
  Constant5/1 -> Max2/2
  Max2/1 -> Product3/2
  Product1/1 -> Prelookup/1  "TurboSpeedNormalized"
  Sqrt/1 -> Product/3, Product6/3
  Add/1 -> Max/1
  Constant2/1 -> Max/2
  Product/1 -> Product1/1  "TurboSpeedReduced"
  InletTemperature_degC/1 -> Add/1
  Constant/1 -> Add/2
